simulink model "plant_setup"  (R2022b)
settings: Solver=VariableStepAuto  StartTime=0.0  StopTime=2.5  RelTol=1e-3
model workspace (MAT data in the model file):
  T_max = Simulink.Parameter
  T_max.Value = 10
  T_max.Description = 'maximum allowable torque command'
  T_max.DataType = 'auto'
  T_max.DocUnits = 'N*m'
  T_max.Complexity = 'real'
  T_max.Dimensions = [1 1]
  bw = Simulink.Parameter
  bw.Value = 0.24
  bw.Description = 'Distance between the two drive wheels'
  bw.DataType = 'auto'
  bw.DocUnits = 'm'
  bw.Complexity = 'real'
  bw.Dimensions = [1 1]
  r_turn = Simulink.Parameter
  r_turn.Value = 0.2
  r_turn.Description = 'Minimum turn radius of the car'
  r_turn.DataType = 'auto'
  r_turn.Min = 0
  r_turn.DocUnits = 'm'
  r_turn.Complexity = 'real'
  r_turn.Dimensions = [1 1]
  r_wheel = Simulink.Parameter
  r_wheel.Value = 0.11
  r_wheel.Description = 'Wheel radius'
  r_wheel.DataType = 'auto'
  r_wheel.DocUnits = 'm'
  r_wheel.Complexity = 'real'
  r_wheel.Dimensions = [1 1]
  v_base = Simulink.Parameter
  v_base.Value = Simulink.data.Expression
  v_base.Value.ExpressionString = "0.12*w_turn_max"
  v_base.Description = 'base wheel speed (m/s) used for turns
    | v_base = w_turn_max 8 bw/2'
  v_base.DataType = 'auto'
  v_base.DocUnits = 'm/s'
  v_base.Complexity = 'real'
  v_base.Dimensions = -1
  v_max = Simulink.Parameter
  v_max.Value = 1
  v_max.Description = 'max car speed in m/s'
  v_max.DataType = 'auto'
  v_max.DocUnits = 'm/s'
  v_max.Complexity = 'real'
  v_max.Dimensions = [1 1]
  w_max = Simulink.Parameter
  w_max.Value = Simulink.data.Expression
  w_max.Value.ExpressionString = "9.0909*v_max"
  w_max.Description = 'max wheel speed in rad/s
    | w_max = v_max/r_wheel'
  w_max.DataType = 'auto'
  w_max.DocUnits = 'rad/s'
  w_max.Complexity = 'real'
  w_max.Dimensions = -1
  w_turn_max = Simulink.Parameter
  w_turn_max.Value = Simulink.data.Expression
  w_turn_max.Value.ExpressionString = "0.45833*w_max"
  w_turn_max.Description = 'max turning speed of car in rad/s
    | w_turn_max = w_max * r_wheel/bw'
  w_turn_max.DataType = 'auto'
  w_turn_max.DocUnits = 'rad/s'
  w_turn_max.Complexity = 'real'
  w_turn_max.Dimensions = -1
undefined symbols (not defined in the file or in its folder): duration, effort, index, joint_name, left_wheel_hinge, model_name, pioneer2dx, right_wheel_hinge
libraries: robotgazebolib x9
settings Model: Creator=22546723@sun.ac.za  LastModifiedBy=22546723@sun.ac.za

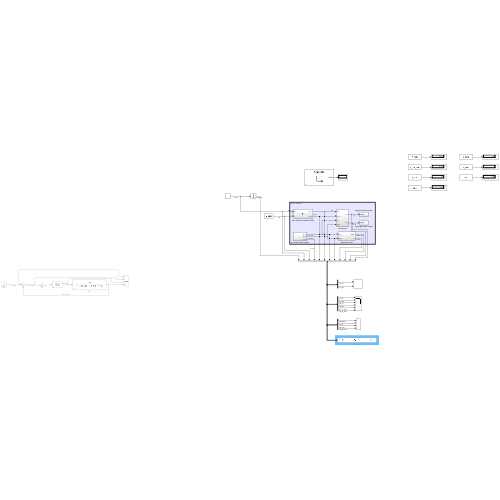
[thumbnail: Simulink's stored preview of the top-level diagram]
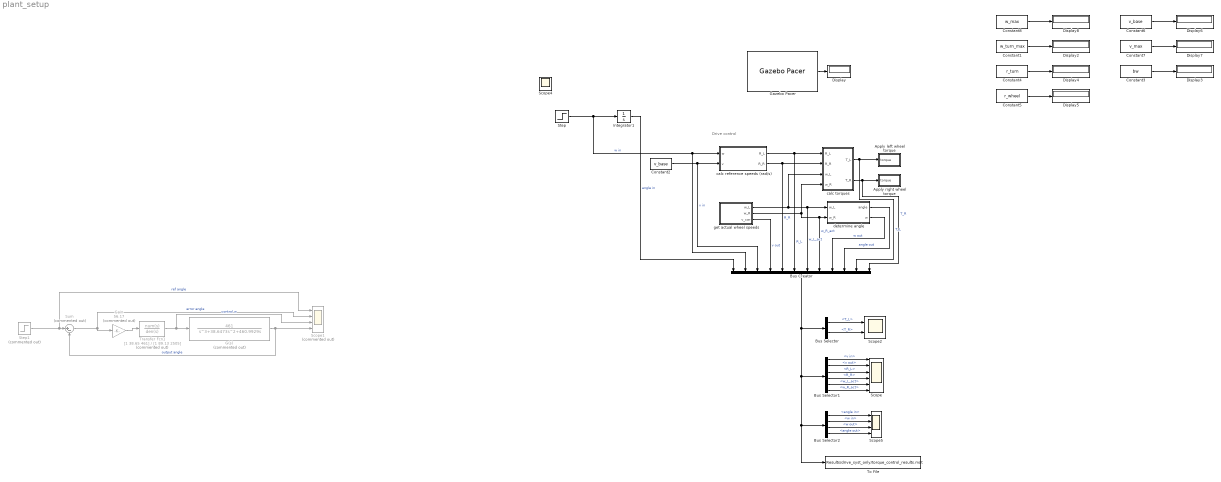
== system plant_setup ==
  note: Drive control
  Apply left wheel torque : Subsystem
  Apply right wheel torque : Subsystem
  Bus Creator : BusCreator  Inputs=12
  Bus Selector : BusSelector  OutputSignals=T_L,T_R
  Bus Selector1 : BusSelector  OutputSignals=v in,v out,R_L,R_R,w_L_act,w_R_act
  Bus Selector2 : BusSelector  OutputSignals=angle in,w in,w out,angle out
  Constant1 : Constant  Value=w_turn_max
  Constant2 : Constant  Value=v_base
  Constant3 : Constant  Value=bw
  Constant4 : Constant  Value=r_turn
  Constant5 : Constant  Value=r_wheel
  Constant6 : Constant  Value=v_base
  Constant7 : Constant  Value=v_max
  Constant8 : Constant  Value=w_max
  Display{,2..8} (8 alike) : Display
  G(s) : TransferFcn  Commented=on  Numerator=461  Denominator="[1   38.6473  460.9929 0]"
  Gain : Gain  Commented=on  Gain=56.17
  Gazebo Pacer : robotgazebolib/Gazebo Pacer  ResetBehavior=Reset Gazebo simulation time  SampleTime=0.001
  Integrator1 : Integrator
  Scope : Scope  NumInputPorts=6
  Scope1 : Scope  Commented=on  NumInputPorts=4
  Scope2 : Scope  NumInputPorts=2
  Scope5 : Scope  NumInputPorts=4
  Step : Step  SampleTime=0
  Step1 : Step  Commented=on  SampleTime=0
  Sum : Sum  Commented=on  Inputs=|+-
  To File : ToFile  Filename=Results/drive_syst_only/torque_control_results.mat  MatrixName=data  SaveFormat=Timeseries
  Transfer Fcn1 : TransferFcn  Commented=on  Numerator=[1 38.65 461]  Denominator=[1 89.13 2505]
  calc reference speeds (rad/s) : Subsystem
  calc torques : Subsystem
  determine angle : Subsystem
  get actual wheel speeds : Subsystem
  Scope4 : Scope
  wires:
  Gazebo Pacer/1 -> Display/1
  Constant2/1 -> calc reference speeds (rad/s)/2(v), Bus Creator/3  "v in"
  calc torques/1(T_L) -> Apply left wheel torque/1(torque), Bus Creator/11  "T_L"
  calc torques/2(T_R) -> Bus Creator/12, Apply right wheel torque/1(torque)  "T_R"
  get actual wheel speeds/1(w_L) -> Bus Creator/7, determine angle/1(w_L), calc torques/3(w_L)  "w_L_act"
  get actual wheel speeds/2(w_R) -> Bus Creator/8, determine angle/2(w_R), calc torques/4(w_R)  "w_R_act"
  determine angle/2(w) -> Bus Creator/9  "w out"
  determine angle/1(angle) -> Bus Creator/10  "angle out"
  Bus Creator/1 -> Bus Selector/1, Bus Selector1/1, Bus Selector2/1, To File/1
  Bus Selector/1 -> Scope2/1  "<T_L>"
  Bus Selector/2 -> Scope2/2  "<T_R>"
  Bus Selector1/3 -> Scope/3  "<R_L>"
  Bus Selector1/4 -> Scope/4  "<R_R>"
  Bus Selector1/5 -> Scope/5  "<w_L_act>"
  Bus Selector1/6 -> Scope/6  "<w_R_act>"
  Transfer Fcn1/1 -> G(s)/1, Scope1/3  "control w"
  Step1/1 -> Scope1/1, Sum/1  "ref angle"
  Sum/1 -> Gain/1, Scope1/2  "error angle"
  G(s)/1 -> Scope1/4, Sum/2  "output angle"
  calc reference speeds (rad/s)/1(R_L) -> calc torques/1(R_L), Bus Creator/6  "R_L"
  calc reference speeds (rad/s)/2(R_R) -> calc torques/2(R_R), Bus Creator/5  "R_R"
  Step/1 -> calc reference speeds (rad/s)/1(w), Bus Creator/2, Integrator1/1  "w in"
  Integrator1/1 -> Bus Creator/1  "angle in"
  Bus Selector2/1 -> Scope5/1  "<angle in>"
  Bus Selector2/2 -> Scope5/2  "<w in>"
  Bus Selector2/3 -> Scope5/3  "<w out>"
  Bus Selector2/4 -> Scope5/4  "<angle out>"
  Gain/1 -> Transfer Fcn1/1
  Constant1/1 -> Display2/1
  Constant3/1 -> Display3/1
  Constant4/1 -> Display4/1
  Constant5/1 -> Display5/1
  Constant6/1 -> Display6/1
  Constant7/1 -> Display7/1
  Constant8/1 -> Display8/1
  Bus Selector1/2 -> Scope/2  "<v out>"
  Bus Selector1/1 -> Scope/1  "<v in>"
  get actual wheel speeds/3(v_car) -> Bus Creator/4  "v out"

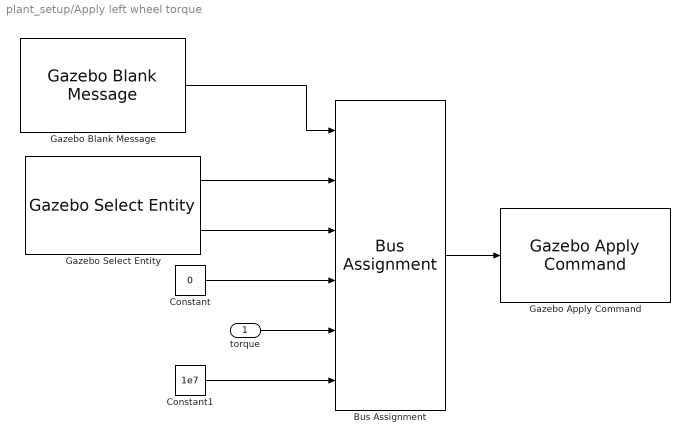
== system plant_setup/Apply left wheel torque ==
  torque : Inport  SampleTime=0.001
  Bus Assignment : BusAssignment  AssignedSignals=model_name,joint_name,index,effort,duration.nano_seconds
  Constant : Constant  Value=0  OutDataTypeStr=uint32  SampleTime=0.001
  Constant1 : Constant  Value=1e7  SampleTime=0.001
  Gazebo Apply Command : robotgazebolib/Gazebo Apply Command  cmdType=ApplyJointTorque  sampleTime=0.001
  Gazebo Blank Message : robotgazebolib/Gazebo Blank Message  msgType=ApplyJointTorque  sampleTime=0.001  busName='Gazebo_SL_Bus_gazebo_msgs_ApplyJointTorque'
  Gazebo Select Entity : robotgazebolib/Gazebo Select Entity  modelElemName=pioneer2dx/left_wheel_hinge  outputArraySize=128  OutputLabel=Joint  SelectType=Joint
  wires:
  Gazebo Select Entity/1 -> Bus Assignment/2
  Bus Assignment/1 -> Gazebo Apply Command/1
  Gazebo Blank Message/1 -> Bus Assignment/1
  Constant/1 -> Bus Assignment/4
  Gazebo Select Entity/2 -> Bus Assignment/3
  Constant1/1 -> Bus Assignment/6
  torque/1 -> Bus Assignment/5

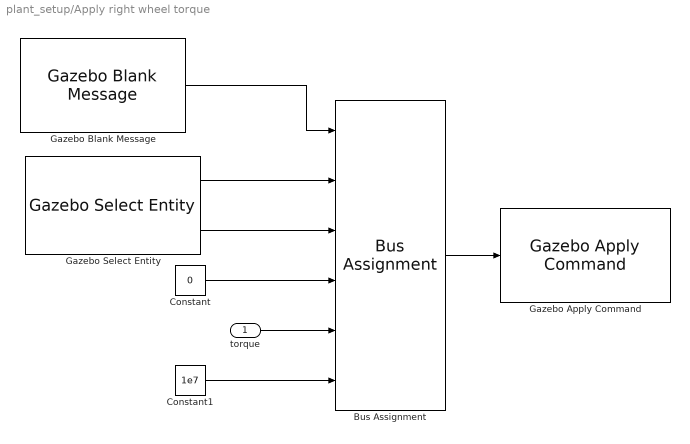
== system plant_setup/Apply right wheel torque ==
  torque : Inport  SampleTime=0.001
  Bus Assignment : BusAssignment  AssignedSignals=model_name,joint_name,index,effort,duration.nano_seconds
  Constant : Constant  Value=0  OutDataTypeStr=uint32  SampleTime=0.001
  Constant1 : Constant  Value=1e7  SampleTime=0.001
  Gazebo Apply Command : robotgazebolib/Gazebo Apply Command  cmdType=ApplyJointTorque  sampleTime=0.001
  Gazebo Blank Message : robotgazebolib/Gazebo Blank Message  msgType=ApplyJointTorque  sampleTime=0.001  busName='Gazebo_SL_Bus_gazebo_msgs_ApplyJointTorque'
  Gazebo Select Entity : robotgazebolib/Gazebo Select Entity  modelElemName=pioneer2dx/right_wheel_hinge  outputArraySize=128  OutputLabel=Joint  SelectType=Joint
  wires:
  Gazebo Select Entity/1 -> Bus Assignment/2
  Bus Assignment/1 -> Gazebo Apply Command/1
  Gazebo Blank Message/1 -> Bus Assignment/1
  Constant/1 -> Bus Assignment/4
  Gazebo Select Entity/2 -> Bus Assignment/3
  Constant1/1 -> Bus Assignment/6
  torque/1 -> Bus Assignment/5

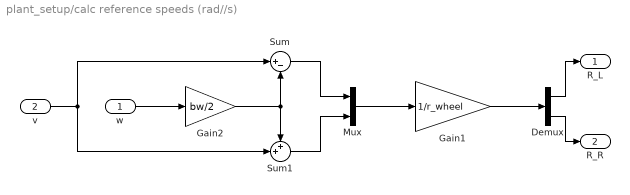
== system plant_setup/calc reference speeds (rad//s) ==
  w : Inport
  v : Inport  Port=2
  Demux : Demux  Outputs=2
  Gain1 : Gain  Gain=1/r_wheel
  Gain2 : Gain  Gain=bw/2
  Mux : Mux  Inputs=2
  Sum : Sum  Inputs=|+-
  Sum1 : Sum  Inputs=++|
  R_L : Outport
  R_R : Outport  Port=2
  wires:
  v/1 -> Sum/1, Sum1/2
  Sum/1 -> Mux/1
  Demux/1 -> R_L/1
  Gain2/1 -> Sum1/1, Sum/2
  Sum1/1 -> Mux/2
  Gain1/1 -> Demux/1
  Mux/1 -> Gain1/1
  w/1 -> Gain2/1
  Demux/2 -> R_R/1

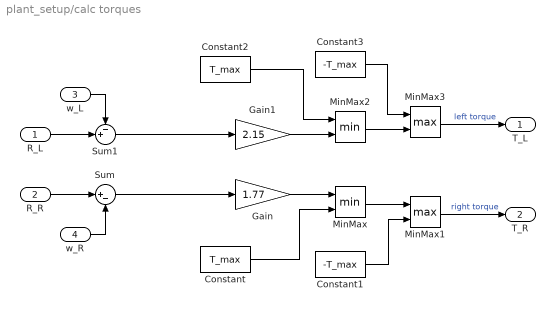
== system plant_setup/calc torques ==
  R_L : Inport
  R_R : Inport  Port=2
  w_L : Inport  Port=3
  w_R : Inport  Port=4
  Constant : Constant  Value=T_max
  Constant1 : Constant  Value=-T_max
  Constant2 : Constant  Value=T_max
  Constant3 : Constant  Value=-T_max
  Gain : Gain  Gain=1.77
  Gain1 : Gain  Gain=2.15
  MinMax : MinMax  Inputs=2
  MinMax1 : MinMax  Function=max  Inputs=2
  MinMax2 : MinMax  Inputs=2
  MinMax3 : MinMax  Function=max  Inputs=2
  Sum : Sum  Inputs=|+-
  Sum1 : Sum  Inputs=-+|
  T_L : Outport
  T_R : Outport  Port=2
  wires:
  Sum/1 -> Gain/1
  w_R/1 -> Sum/2
  Sum1/1 -> Gain1/1
  R_R/1 -> Sum/1
  w_L/1 -> Sum1/1
  R_L/1 -> Sum1/2
  Gain/1 -> MinMax/1
  Constant/1 -> MinMax/2
  MinMax/1 -> MinMax1/1
  Constant1/1 -> MinMax1/2
  Gain1/1 -> MinMax2/2
  Constant2/1 -> MinMax2/1
  MinMax2/1 -> MinMax3/2
  Constant3/1 -> MinMax3/1
  MinMax3/1 -> T_L/1  "left torque"
  MinMax1/1 -> T_R/1  "right torque"

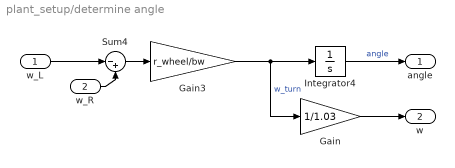
== system plant_setup/determine angle ==
  w_L : Inport
  w_R : Inport  Port=2
  Gain : Gain  Gain=1/1.03
  Gain3 : Gain  Gain=r_wheel/bw
  Integrator4 : Integrator
  Sum4 : Sum  Inputs=|-+
  angle : Outport
  w : Outport  Port=2
  wires:
  Gain3/1 -> Gain/1, Integrator4/1  "w_turn"
  Sum4/1 -> Gain3/1
  w_R/1 -> Sum4/2
  Integrator4/1 -> angle/1  "angle"
  w_L/1 -> Sum4/1
  Gain/1 -> w/1

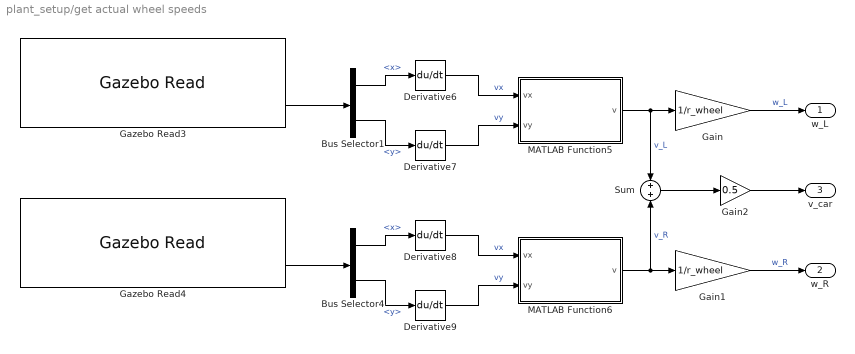
== system plant_setup/get actual wheel speeds ==
  Bus Selector1 : BusSelector  OutputSignals=position.x,position.y
  Bus Selector4 : BusSelector  OutputSignals=position.x,position.y
  Derivative{6..9} (4 alike) : Derivative
  Gain : Gain  Gain=1/r_wheel
  Gain1 : Gain  Gain=1/r_wheel
  Gain2 : Gain  Gain=0.5
  Gazebo Read3 : robotgazebolib/Gazebo Read  topicSource=From Gazebo  topic=/gazebo/ground_truth/world_pose/pioneer2dx/left_wheel  messageType=gazebo_msgs/Pose  sampleTime=0.001  fixedAxisBusStatus=off  jointAxisCount=2
  Gazebo Read4 : robotgazebolib/Gazebo Read  topicSource=From Gazebo  topic=/gazebo/ground_truth/world_pose/pioneer2dx/right_wheel  messageType=gazebo_msgs/Pose  sampleTime=0.001  fixedAxisBusStatus=off  jointAxisCount=2
  MATLAB Function5 : MATLAB Function  TreatAsAtomicUnit=on
  MATLAB Function6 : MATLAB Function  TreatAsAtomicUnit=on
  Sum : Sum  Inputs=+|+
  w_L : Outport
  w_R : Outport  Port=2
  v_car : Outport  Port=3
  wires:
  Bus Selector4/1 -> Derivative8/1  "<x>"
  Bus Selector4/2 -> Derivative9/1  "<y>"
  Derivative8/1 -> MATLAB Function6/1(vx)  "vx"
  Derivative9/1 -> MATLAB Function6/2(vy)  "vy"
  Derivative6/1 -> MATLAB Function5/1(vx)  "vx"
  Gazebo Read3/2 -> Bus Selector1/1
  Bus Selector1/1 -> Derivative6/1  "<x>"
  Bus Selector1/2 -> Derivative7/1  "<y>"
  Gazebo Read4/2 -> Bus Selector4/1
  Derivative7/1 -> MATLAB Function5/2(vy)  "vy"
  MATLAB Function5/1(v) -> Sum/1, Gain/1  "v_L"
  Gain/1 -> w_L/1  "w_L"
  MATLAB Function6/1(v) -> Sum/2, Gain1/1  "v_R"
  Gain1/1 -> w_R/1  "w_R"
  Sum/1 -> Gain2/1
  Gain2/1 -> v_car/1

== matlab function plant_setup/get actual wheel speeds/MATLAB Function6 ==
  settings: updateMethod=DISCRETE
  data: vx input; v output; vy input
function v = detSpeed(vx, vy)
persistent prev_x
persistent prev_y

if isempty(prev_x)
    prev_x = 0;
end

if isempty(prev_y)
    prev_y = 0;
end

if abs(prev_x - vx)>1
    vx = prev_x;
else
    prev_x = vx;
end

if abs(prev_y - vy)>1
    vy = prev_y;
else 
    prev_y = vy;
end

v = sqrt(vx^2 + vy^2);

== matlab function plant_setup/get actual wheel speeds/MATLAB Function5 ==
  settings: updateMethod=DISCRETE
  data: vx input; v output; vy input
function v = detSpeed(vx, vy)
persistent prev_x
persistent prev_y

if isempty(prev_x)
    prev_x = 0;
end

if isempty(prev_y)
    prev_y = 0;
end

if abs(prev_x - vx)>1
    vx = prev_x;
else
    prev_x = vx;
end

if abs(prev_y - vy)>1
    vy = prev_y;
else 
    prev_y = vy;
end

v = sqrt(vx^2 + vy^2);
